simulink library "APPS_BSPC"  (R2024a)
settings: Solver=VariableStepAuto  StartTime=0.0  StopTime=10.0  RelTol=1e-3
undefined symbols (not defined in the file or in its folder): raptor_xcp_function
libraries: Raptor_lib x7, Utilities x4, simulink x2
settings Model: Creator=serga  LastModifiedBy=serga

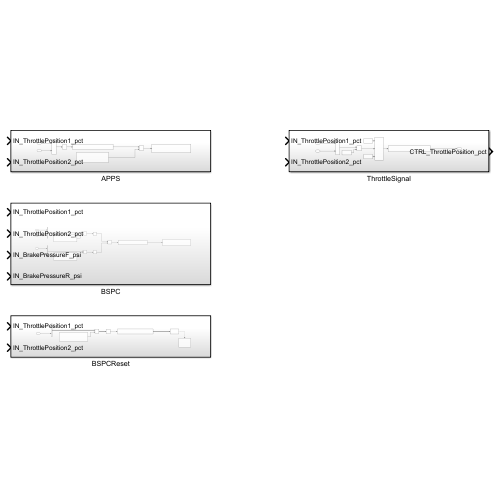
[thumbnail: Simulink's stored preview of the top-level diagram]
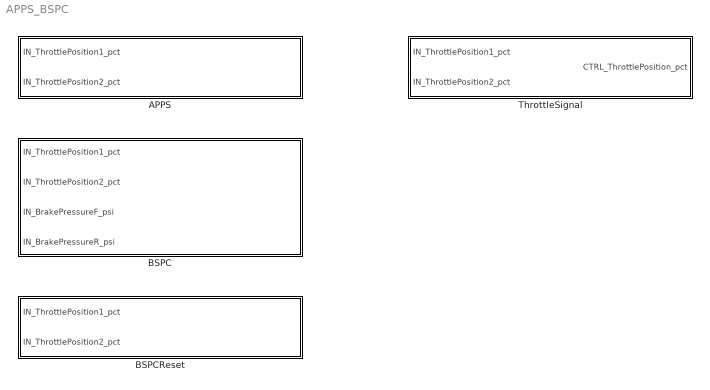
== system APPS_BSPC ==
  APPS : Subsystem
  BSPC : Subsystem
  BSPCReset : Subsystem
  ThrottleSignal : Subsystem

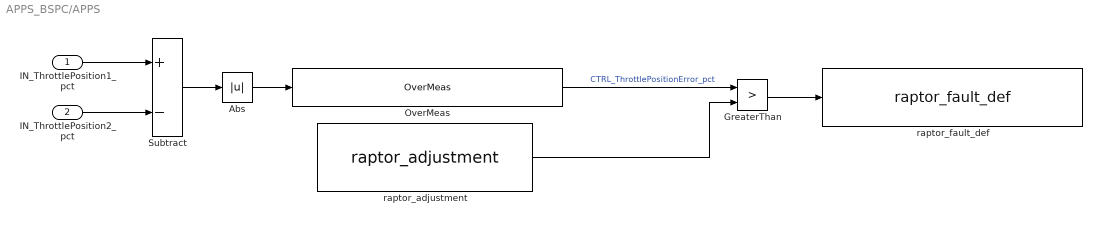
== system APPS_BSPC/APPS ==
  IN_ThrottlePosition1_pct : Inport
  IN_ThrottlePosition2_pct : Inport  Port=2
  Abs : Abs  SaturateOnIntegerOverflow=off
  GreaterThan : RelationalOperator  Operator=>  OutDataTypeStr=boolean  RndMeth=Simplest  InputSameDT=off
  OverMeas : Utilities/OverMeas  sigName='CTRL_ThrottlePositionError_pct'  min=0  max=100
  Subtract : Sum  Inputs=+-
  raptor_adjustment : Raptor_lib/Data Storage/raptor_adjustment  paramName='CTRL_APPSThresh_pct'  nameSource=Parameter  initValue=10  dataType=single  storage=Calibration  calDispType=Number  calEnum={'False', 'True'}  calGain=1.0  calOffset=0.0  calMax=100  calMin=0  calFormat='-1'  calUnit=''  calHelp=''  calAccess=1  calFunction=raptor_xcp_function(gcb)  calDispHeaders=off  calColHeaders={'Col1' 'Col2' 'Col3'}  calRowHeaders={'Row1' 'Row2' 'Row3'}
      settings: SourceProductName=Raptor
  raptor_fault_def : Raptor_lib/Faults/raptor_fault_def  faultName='CTRL_APPSFault'  persist=on  sticky=off  emisRelated=off  singleTrip=off  clearMethod=Standard  xLimit=25  yLimit=50  calEnable=on  addDisable=off  calAccess=1  calFunction='System | FaultManager'
      settings: SourceProductName=Raptor
  wires:
  IN_ThrottlePosition1_pct/1 -> Subtract/1
  IN_ThrottlePosition2_pct/1 -> Subtract/2
  Subtract/1 -> Abs/1
  Abs/1 -> OverMeas/1
  raptor_adjustment/1 -> GreaterThan/2
  GreaterThan/1 -> raptor_fault_def/1
  OverMeas/1 -> GreaterThan/1  "CTRL_ThrottlePositionError_pct"

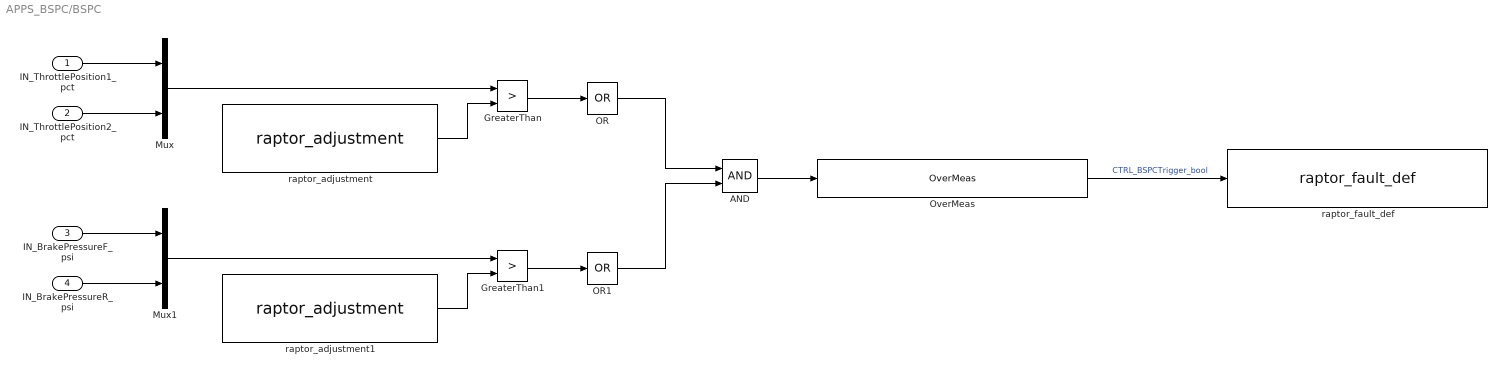
== system APPS_BSPC/BSPC ==
  IN_ThrottlePosition1_pct : Inport
  IN_ThrottlePosition2_pct : Inport  Port=2
  IN_BrakePressureF_psi : Inport  Port=3
  IN_BrakePressureR_psi : Inport  Port=4
  AND : Logic  AllPortsSameDT=off  OutDataTypeStr=boolean
  GreaterThan : RelationalOperator  Operator=>  OutDataTypeStr=boolean  RndMeth=Simplest  InputSameDT=off
  GreaterThan1 : RelationalOperator  Operator=>  OutDataTypeStr=boolean  RndMeth=Simplest  InputSameDT=off
  Mux : Mux  Inputs=2
  Mux1 : Mux  Inputs=2
  OR : Logic  Operator=OR  Inputs=1  AllPortsSameDT=off  OutDataTypeStr=boolean
  OR1 : Logic  Operator=OR  Inputs=1  AllPortsSameDT=off  OutDataTypeStr=boolean
  OverMeas : Utilities/OverMeas  sigName='CTRL_BSPCTrigger_bool'  min=0  max=1
  raptor_adjustment : Raptor_lib/Data Storage/raptor_adjustment  paramName='CTRL_BSPCThrottleThresh_pct'  nameSource=Parameter  initValue=25  dataType=single  storage=Calibration  calDispType=Number  calEnum={'False', 'True'}  calGain=1.0  calOffset=0.0  calMax=100  calMin=0  calFormat='-1'  calUnit=''  calHelp=''  calAccess=1  calFunction=raptor_xcp_function(gcb)  calDispHeaders=off  calColHeaders={'Col1' 'Col2' 'Col3'}  calRowHeaders={'Row1' 'Row2' 'Row3'}
      settings: SourceProductName=Raptor
  raptor_adjustment1 : Raptor_lib/Data Storage/raptor_adjustment  paramName='CTRL_BSPCBrakeThresh_psi'  nameSource=Parameter  initValue=150  dataType=single  storage=Calibration  calDispType=Number  calEnum={'False', 'True'}  calGain=1.0  calOffset=0.0  calMax=2000  calMin=0  calFormat='-1'  calUnit=''  calHelp=''  calAccess=1  calFunction=raptor_xcp_function(gcb)  calDispHeaders=off  calColHeaders={'Col1' 'Col2' 'Col3'}  calRowHeaders={'Row1' 'Row2' 'Row3'}
      settings: SourceProductName=Raptor
  raptor_fault_def : Raptor_lib/Faults/raptor_fault_def  faultName='CTRL_BSPCTriggerFault'  persist=off  sticky=on  emisRelated=off  singleTrip=off  clearMethod=Standard  xLimit=25  yLimit=50  calEnable=on  addDisable=off  calAccess=1  calFunction='System | FaultManager'
      settings: SourceProductName=Raptor
  wires:
  IN_ThrottlePosition1_pct/1 -> Mux/1
  IN_ThrottlePosition2_pct/1 -> Mux/2
  Mux/1 -> GreaterThan/1
  raptor_adjustment/1 -> GreaterThan/2
  IN_BrakePressureR_psi/1 -> Mux1/2
  IN_BrakePressureF_psi/1 -> Mux1/1
  Mux1/1 -> GreaterThan1/1
  raptor_adjustment1/1 -> GreaterThan1/2
  GreaterThan/1 -> OR/1
  GreaterThan1/1 -> OR1/1
  OR/1 -> AND/1
  OR1/1 -> AND/2
  AND/1 -> OverMeas/1
  OverMeas/1 -> raptor_fault_def/1  "CTRL_BSPCTrigger_bool"

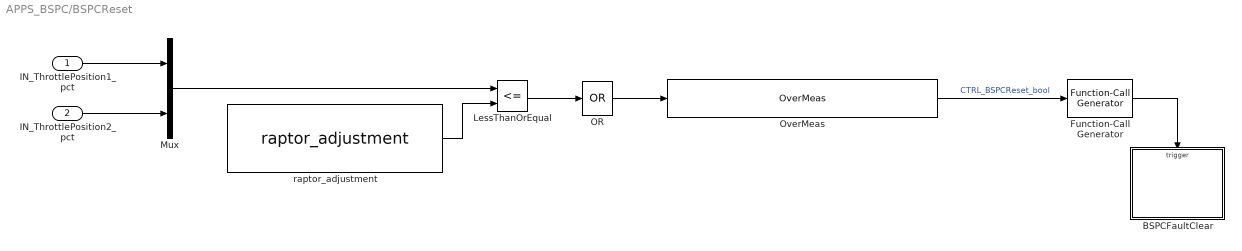
== system APPS_BSPC/BSPCReset ==
  IN_ThrottlePosition1_pct : Inport
  IN_ThrottlePosition2_pct : Inport  Port=2
  BSPCFaultClear : Subsystem  TreatAsAtomicUnit=on
  Function-Call Generator : simulink/Ports & Subsystems/Function-Call Generator  sample_time=1  numberOfIterations=1  DisallowWideOutput=off  ShowEnablePort=on
  LessThanOrEqual : RelationalOperator  Operator=<=  OutDataTypeStr=boolean  RndMeth=Simplest  InputSameDT=off
  Mux : Mux  Inputs=2
  OR : Logic  Operator=OR  Inputs=1  AllPortsSameDT=off  OutDataTypeStr=boolean
  OverMeas : Utilities/OverMeas  sigName='CTRL_BSPCReset_bool'  min=0  max=1
  raptor_adjustment : Raptor_lib/Data Storage/raptor_adjustment  paramName='CTRL_BSPCResetThresh_pct'  nameSource=Parameter  initValue=5  dataType=single  storage=Calibration  calDispType=Number  calEnum={'False', 'True'}  calGain=1.0  calOffset=0.0  calMax=100  calMin=0  calFormat='-1'  calUnit=''  calHelp=''  calAccess=1  calFunction=raptor_xcp_function(gcb)  calDispHeaders=off  calColHeaders={'Col1' 'Col2' 'Col3'}  calRowHeaders={'Row1' 'Row2' 'Row3'}
      settings: SourceProductName=Raptor
  wires:
  OR/1 -> OverMeas/1
  IN_ThrottlePosition1_pct/1 -> Mux/1
  IN_ThrottlePosition2_pct/1 -> Mux/2
  Mux/1 -> LessThanOrEqual/1
  raptor_adjustment/1 -> LessThanOrEqual/2
  LessThanOrEqual/1 -> OR/1
  OverMeas/1 -> Function-Call Generator/1  "CTRL_BSPCReset_bool"
  Function-Call Generator/1 -> BSPCFaultClear/Trigger

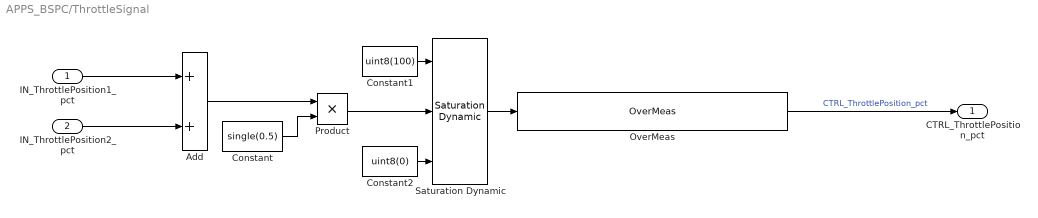
== system APPS_BSPC/ThrottleSignal ==
  IN_ThrottlePosition1_pct : Inport
  IN_ThrottlePosition2_pct : Inport  Port=2
  Add : Sum
  Constant : Constant  Value=single(0.5)
  Constant1 : Constant  Value=uint8(100)
  Constant2 : Constant  Value=uint8(0)
  OverMeas : Utilities/OverMeas  sigName='CTRL_ThrottlePosition_pct'  min=0  max=100
  Product : Product
  Saturation Dynamic : simulink/Discontinuities/Saturation Dynamic  OutMin=[]  OutMax=[]  OutDataTypeStr=Inherit: Same as second input  OutDataType=fixdt(1, 16)  OutScaling=2^-10  DoSatur=off
  CTRL_ThrottlePosition_pct : Outport
  wires:
  IN_ThrottlePosition1_pct/1 -> Add/1
  IN_ThrottlePosition2_pct/1 -> Add/2
  Add/1 -> Product/1
  Constant/1 -> Product/2
  Product/1 -> Saturation Dynamic/2
  OverMeas/1 -> CTRL_ThrottlePosition_pct/1  "CTRL_ThrottlePosition_pct"
  Saturation Dynamic/1 -> OverMeas/1
  Constant1/1 -> Saturation Dynamic/1
  Constant2/1 -> Saturation Dynamic/3

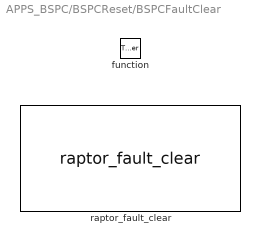
== system APPS_BSPC/BSPCReset/BSPCFaultClear ==
  function : TriggerPort  TriggerType=function-call  VariantControl=(inherit)
  raptor_fault_clear : Raptor_lib/Faults/raptor_fault_clear  faultSource=Parameter  faultName='CTRL_BSPCTriggerFault'
      settings: SourceProductName=Raptor
